simulink model "MSD_NL_Javi_fix"  (R2023b)
settings: Solver=ode4  StartTime=0.0  StopTime=Tf  FixedStep=dt  MaxStep=0.1  RelTol=1e-3
undefined symbols (not defined in the file): b1, b2, F, k1, k2, M, m, U0
settings Model: Creator=The MathWorks, Inc.  LastModifiedBy=E. Javier Olucha
settings DebuggingCC: UnconnectedInputMsg=warning  UnconnectedOutputMsg=warning  UnconnectedLineMsg=warning  SubsystemReferenceDiagnosticForUnitTest=warning
settings ModelReferenceCC: EnableRefExpFcnMdlSchedulingChecks=on
settings RTWCC: DLArmComputeVersion=19.05

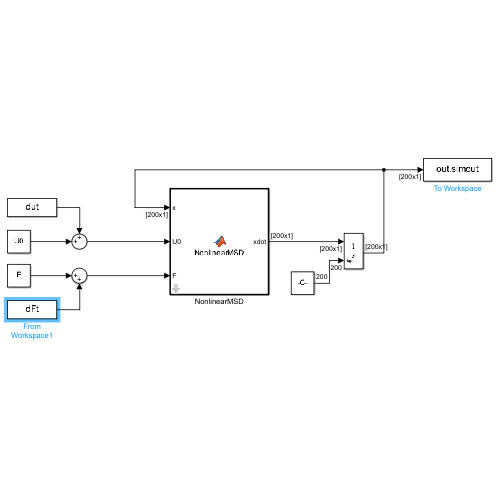
[thumbnail: Simulink's stored preview of the top-level diagram]
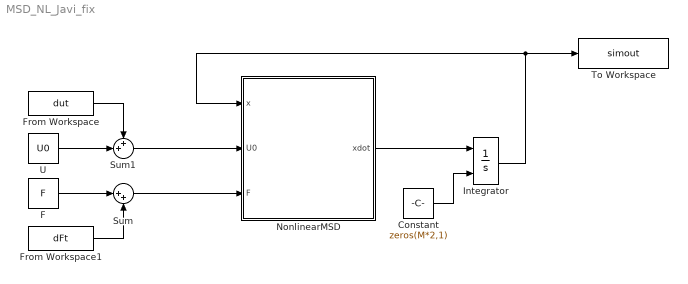
== system MSD_NL_Javi_fix ==
  Constant : Constant  Value=zeros(M*2,1)
  F : Constant  Value=F
  From Workspace : FromWorkspace  VariableName=dut
  From Workspace1 : FromWorkspace  VariableName=dFt  Interpolate=off  OutputAfterFinalValue=Holding final value
  Integrator : Integrator  InitialConditionSource=external
  NonlinearMSD : MATLAB Function  TreatAsAtomicUnit=on  mask{m=m, k1=k1, k2=k2, b1=b1, b2=b2}
      mask prompts: m "mass"
  Sum : Sum  Inputs=|++
  Sum1 : Sum  Inputs=++|
  To Workspace : ToWorkspace  VariableName=simout  SaveFormat=Timeseries  SampleTime=-1
  U : Constant  Value=U0
  wires:
  Constant/1 -> Integrator/2
  NonlinearMSD/1(xdot) -> Integrator/1
  F/1 -> Sum/1
  U/1 -> Sum1/2
  Sum/1 -> NonlinearMSD/3(F)
  From Workspace1/1 -> Sum/2
  Sum1/1 -> NonlinearMSD/2(U0)
  From Workspace/1 -> Sum1/1
  Integrator/1 -> To Workspace/1, NonlinearMSD/1(x)

== matlab function MSD_NL_Javi_fix/NonlinearMSD ==
  data: x input; m parameter; xdot output; k1 parameter; k2 parameter; b1 parameter; b2 parameter; U0 input; F input
function xdot = NonlinearMSD(x, m, k1, k2, b1, b2, U0, F)
% function xdot = NonlinearMSD(t,x,m,k1,k2,b1,b2,F,u)
% 
% This function implements the ordinary differential equation for the
% nonlinear mass-spring-damper system.  The system consists of M blocks 
% connected by nonlinear springs and dampers.  In addition, each block
% is connected to a wall by a nonlinear spring and damper. The system has 
% an input force u and an exogeneous force F on the M^th block.
%
% Inputs:
%  *t = time, sec
%  *x = 2M-by-1 vector specifying the state of the M block, nonlinear 
%       mass-spring-damper system as:
%          x = [p1; p2; ...; pM; v1; v2;....; vM]
%       where (pi,vi) are the position (m) and velocity (m/s) of block i.
%  *m = Mass of individual blocks, kg
%  *k1 = Linear spring constant, N/m
%  *k2 = Cubic spring constant, N/m^3
%  *b1 = Linear damping constant, N/(m/s)
%  *b2 = Cubic damping constant, N/(m/s)^3
%  *F = Nf-by-2 matrix specifying the force (in N) on the M^th block. 
%       The i^th row of F specifies a time F(i,1) and force F(i,2). The
%       force applied at time t in the simulation is computed by 
%       interpolating this matrix of data.
%  *u = Nu-by-2 matrix specifying the force (in N) on the M^th block.
%       The i^th row of u specifies a time u(i,1) and force u(i,2). 
%       The force applied at time t in the simulation is computed by 
%       interpolating this matrix of data.
%
% Output:
%  *xdot = 2M-by-1 vector specifying the derivative of the system:
%          xdot = [v1; v2;....; vM; a1; a2; ...; aM]
%       where (vi,ai) are the velocity (m/s) and acceleration (m/s^2)
%       of block i.
%

% # of Masses
M = numel(x)/2;
xdot = zeros(2*M,1);

% Extract positions and velocities
p = x(1:M);
v = x(M+1:end);

% Compute the block accelerations
a = zeros(M,1);
for i=1:M
    if i==1 && M==1
        % Special Case: Only a single block
        % Total force on mass
        Ftot = U0 + F;        
    elseif i==1                        
        % Total force on mass
        Ftot = Fs(p(2)-p(1),k1,k2) + Fd(v(2)-v(1),b1,b2);
    elseif i==M
        % Total force on mass
        Ftot = U0 + F - Fs(p(M)-p(M-1),k1,k2) - Fd(v(M)-v(M-1),b1,b2);
    else       
        % Total force on mass
        Ftot = - Fs(p(i)-p(i-1),k1,k2) - Fd(v(i)-v(i-1),b1,b2) ...
                + Fs(p(i+1)-p(i),k1,k2) + Fd(v(i+1)-v(i),b1,b2);
    end
    
    % Connect each block by an additional spring/damper to wall
    Ftot = Ftot - Fs(p(i),k1,k2) - Fd(v(i),b1,b2);
    
    % Acceleration
    a(i) = Ftot/m;
end

% State derivative 
xdot = [v; a];



%% Local function to compute spring force
function y = Fs(u,k1,k2)
y = k1*u+k2*u^3;

%% Local function to compute damping force
function y = Fd(u,b1,b2)
y = b1*u+b2*u^3;
